simulink model "pdl_linear_hw4non"  (R2017a)
settings: Solver=VariableStepAuto  StartTime=0.0  StopTime=duration  FixedStep=Ts  RelTol=1e-3
values from neighbouring files (symbols this model uses):
  A = [0 0 1 0; 0 0 0 1; -k/M -m*g/M -b/M 0; k/(M*L) (m+M)*g/(M*L) b/(M*L) 0]    [pendulum_hw4non.m]
  B = [0;0;1/M;-1/(M*L)]    [pendulum_hw4non.m]
  C = [1 0 0 0; 0 1 0 0]    [pendulum_hw4non.m]
  E = [0 0;0 0;-1/M 0;1/(M*L) -1/(m*L)]    [pendulum_hw4non.m]
  f_p = 1e-4    (= 0.0001)    [pendulum_hw4non.m]
  m_p = 1e-7    (= 1e-07)    [pendulum_hw4non.m]
  Q_k = diag([1 1])    [pendulum_hw4non.m]
  R_k = 1e-4*diag([1 1])    [pendulum_hw4non.m]
  Ts = 0.001    [pendulum_hw4non.m]
  w_p = 10    [pendulum_hw4non.m]
  X_0 = [0;0*pi/180;0;0]    [pendulum_hw4non.m]
undefined symbols (not defined in the file or in its folder): Delta, Gamma, LC1_D, Phi
libraries: simulink x3, simulink_extras x2
settings Model: Creator=Salmon  LastModifiedBy=Salmon

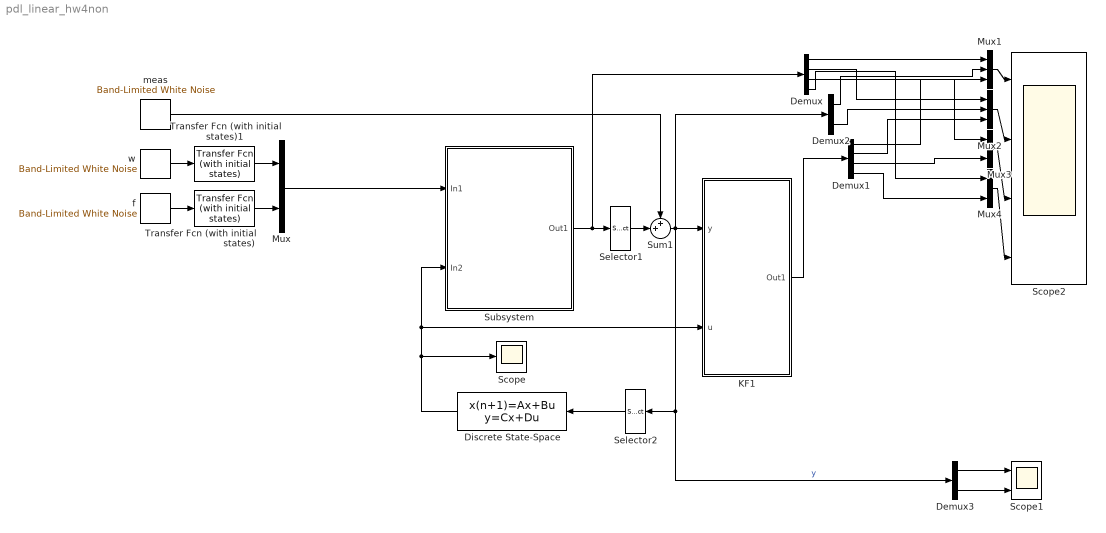
== system pdl_linear_hw4non ==
  Demux : Demux
  Demux1 : Demux
  Demux2 : Demux  Outputs=2
  Demux3 : Demux  Outputs=2
  Discrete State-Space : DiscreteStateSpace  A=LC1_D.A  B=LC1_D.B  C=LC1_D.C  D=LC1_D.D  SampleTime=Ts
  KF1 : Subsystem
  Mux : Mux  Inputs=2
  Mux1 : Mux  Inputs=3
  Mux2 : Mux  Inputs=3
  Mux3 : Mux  Inputs=2
  Mux4 : Mux  Inputs=2
  Scope : Scope
  Scope1 : Scope  NumInputPorts=2
  Scope2 : Scope  NumInputPorts=4
  Selector1 : Selector  InputPortWidth=4  IndexOptions=Index vector (dialog)  Indices=[1 2]  OutputSizes=1
  Selector2 : Selector  InputPortWidth=2  IndexOptions=Index vector (dialog)  Indices=[2 1]  OutputSizes=1
  Subsystem : Subsystem
  Sum1 : Sum  Inputs=++|
  Transfer Fcn (with initial states) : simulink_extras/Additional Linear/Transfer Fcn (with initial states)  N=[0.64]  D="[1  0.8]"  X0=0.5
  Transfer Fcn (with initial states)1 : simulink_extras/Additional Linear/Transfer Fcn (with initial states)  N=[0.64]  D="[1  0.8]"  X0=0.5
  f : simulink/Sources/Band-Limited White Noise  Cov=[f_p]  Ts=Ts  seed=[23341]
  meas : simulink/Sources/Band-Limited White Noise  Cov=[m_p,m_p]  Ts=Ts  seed=[123,23341]
  w : simulink/Sources/Band-Limited White Noise  Cov=[w_p]  Ts=Ts  seed=[23341]
  wires:
  w/1 -> Transfer Fcn (with initial states)1/1
  f/1 -> Transfer Fcn (with initial states)/1
  Mux/1 -> Subsystem/1(In1)
  Subsystem/1(Out1) -> Selector1/1, Demux/1
  Discrete State-Space/1 -> Subsystem/2(In2), KF1/2(u), Scope/1
  Demux/1 -> Mux1/1
  Demux/2 -> Mux2/1
  Demux/3 -> Mux3/1
  Demux/4 -> Mux4/1
  Selector1/1 -> Sum1/2
  Demux1/1 -> Mux1/3
  KF1/1(Out1) -> Demux1/1
  Demux1/3 -> Mux3/2
  Demux1/2 -> Mux2/3
  Demux1/4 -> Mux4/2
  meas/1 -> Sum1/1
  Demux2/1 -> Mux1/2
  Demux2/2 -> Mux2/2
  Mux1/1 -> Scope2/1
  Mux2/1 -> Scope2/2
  Mux3/1 -> Scope2/3
  Mux4/1 -> Scope2/4
  Transfer Fcn (with initial states)1/1 -> Mux/1
  Transfer Fcn (with initial states)/1 -> Mux/2
  Selector2/1 -> Discrete State-Space/1
  Demux3/2 -> Scope1/2
  Demux3/1 -> Scope1/1
  Sum1/1 -> Demux3/1, Selector2/1, Demux2/1, KF1/1(y)  "y"

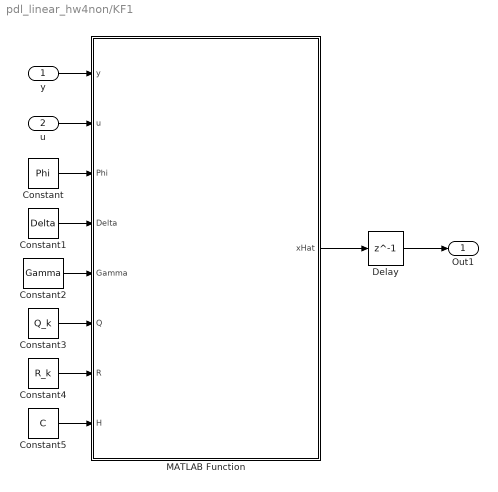
== system pdl_linear_hw4non/KF1 ==
  y : Inport
  u : Inport  Port=2
  Constant : Constant  Value=Phi
  Constant1 : Constant  Value=Delta
  Constant2 : Constant  Value=Gamma
  Constant3 : Constant  Value=Q_k
  Constant4 : Constant  Value=R_k
  Constant5 : Constant  Value=C
  Delay : Delay  DelayLength=1  InitialCondition=0
  MATLAB Function : MATLAB Function  TreatAsAtomicUnit=on
  Out1 : Outport
  wires:
  y/1 -> MATLAB Function/1(y)
  MATLAB Function/1(xHat) -> Delay/1
  u/1 -> MATLAB Function/2(u)
  Constant/1 -> MATLAB Function/3(Phi)
  Constant1/1 -> MATLAB Function/4(Delta)
  Constant3/1 -> MATLAB Function/6(Q)
  Constant2/1 -> MATLAB Function/5(Gamma)
  Constant4/1 -> MATLAB Function/7(R)
  Constant5/1 -> MATLAB Function/8(H)
  Delay/1 -> Out1/1

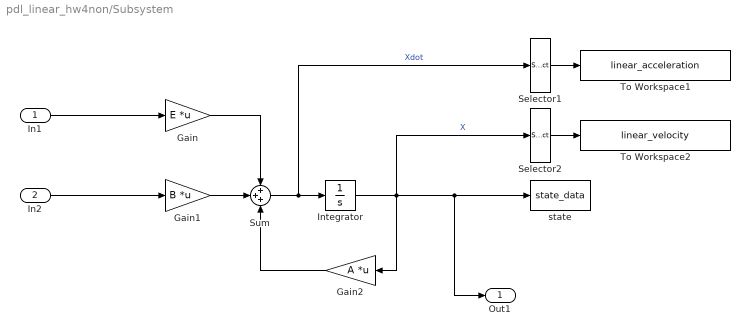
== system pdl_linear_hw4non/Subsystem ==
  In1 : Inport
  In2 : Inport  Port=2
  Gain : Gain  Gain=E  Multiplication=Matrix(K*u)
  Gain1 : Gain  Gain=B  Multiplication=Matrix(K*u)
  Gain2 : Gain  Gain=A  Multiplication=Matrix(K*u)
  Integrator : Integrator  InitialCondition=X_0
  Selector1 : Selector  InputPortWidth=4  IndexOptions=Index vector (dialog)  Indices=[3]  OutputSizes=1
  Selector2 : Selector  InputPortWidth=4  IndexOptions=Index vector (dialog)  Indices=[3]  OutputSizes=1
  Sum : Sum  Inputs=+++
  To Workspace1 : ToWorkspace  VariableName=linear_acceleration  SaveFormat=Structure With Time  SampleTime=-1
  To Workspace2 : ToWorkspace  VariableName=linear_velocity  SaveFormat=Structure With Time  SampleTime=-1
  state : ToWorkspace  VariableName=state_data  SaveFormat=Structure With Time  SampleTime=Ts
  Out1 : Outport
  wires:
  In1/1 -> Gain/1
  Gain/1 -> Sum/1
  Gain1/1 -> Sum/2
  Selector2/1 -> To Workspace2/1
  Selector1/1 -> To Workspace1/1
  Gain2/1 -> Sum/3
  In2/1 -> Gain1/1
  Integrator/1 -> Gain2/1, Selector2/1, Out1/1, state/1  "X"
  Sum/1 -> Integrator/1, Selector1/1  "Xdot"

== matlab function pdl_linear_hw4non/KF1/MATLAB Function ==
  data: y input; u input; xHat output; Phi input; Delta input; Gamma input; Q input; R input; H input
function xHat = fcn(y,u,Phi,Delta,Gamma,Q,R,H)

persistent Pbar xbar

% init. Pbar xbar
if isempty(Pbar)
    Pbar = 1e-6*eye(4);
end

if isempty(xbar)
    xbar = zeros(4,1);
end

% 1. Kalman gain
K = Pbar*H'*[H*Pbar*H'+R]^(-1);

% 2. state est. update
xHat = xbar + K*[y-H*xbar];

% 3. error covariance update
Phat = [eye(4)-K*H]*Pbar*[eye(4)-K*H]'+K*R*K';

% 4. state est. propagation
xbar = Phi*xHat+Delta*u;

% 5. error covariance propagation
Pbar = Phi*Phat*Phi'+Gamma*Q*Gamma';
